simulink model "Upgrade3"  (R2017a)
settings: Solver=FixedStepDiscrete  StartTime=0.0  StopTime=2700000  RelTol=1e-3
model workspace: external: MAT-File upgradeParams.mat (data not in the file)
values from neighbouring files (symbols this model uses):
  ambulance_speed = 60    [upgradeParams.mat]
  delayConstant = 0.25    [upgradeParams.mat]
  hospital_dist = 10    [upgradeParams.mat]
  radius = 15    [upgradeParams.mat]
  transfer_lag = 50    [upgradeParams.mat]
undefined symbols (not defined in the file or in its folder): entity, m, n, readTimer
libraries: sldelib x1
(part 2 of 3)

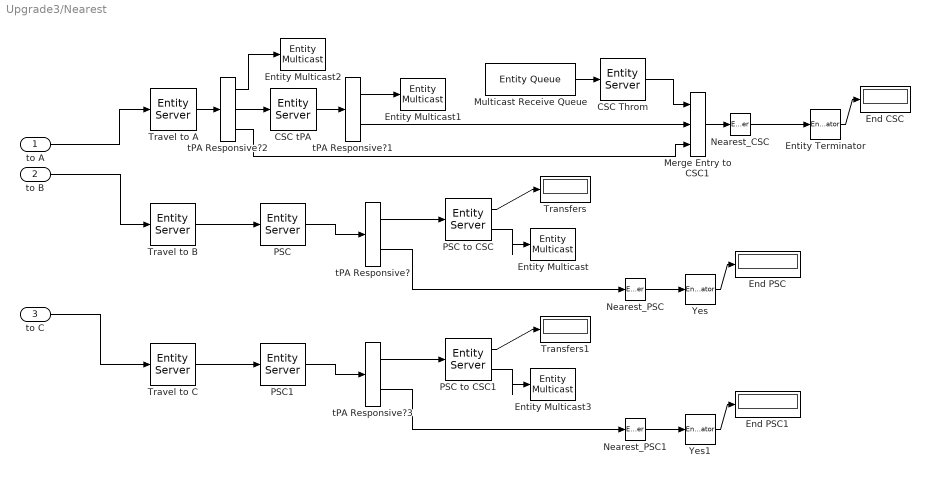
== system Upgrade3/Nearest ==
  to A : Inport
  to B : Inport  Port=2
  to C : Inport  Port=3
  CSC Throm : EntityServer  InputPortMessageModes=m  OutputPortMessageModes=m  Capacity=2  ServiceTimeSource=MATLAB action  ServiceTimeValue=CSC_NTP  ServiceTimeAction=|  ServiceCompleteAction=|
      ServiceTimeAction=|
      | if ~entity.CTA
      |     %did respond to tPA or have hemorrhage
      |     %then only did CTA and discovered no go
      |     if entity.tPA && ((entity.tPAresponse < tPAresp_LVO) | (entity.ICHresp < ICHrate))
      |         dt = CTA_time;
      |     else
      |         dt = CTA_time + CSC_NTP;
      |     end
      | else
      |     dt = CSC_NTP;
      | end
      ServiceCompleteAction=|
      | if ~entity.CTA
      |     entity.CTA=true;
      | end
      | 
      | if entity.throm
      |     %if previously already decided should have thrombectomy
      |     %outcomeType already assigned
      |     entity.thromTime = startTimer() - entity.startTime;
      | elseif ~entity.tPA
      |     %bypassed tPA in CSC
      |     entity.throm = true;
      |     entity.thromTime = startTimer() - entity.startTime;
      |     entity.outcomeType = 3;
      | elseif (entity.tPAresponse >= tPAresp_LVO) && (entity.ICHresp > ICHrate)
      |     %did not respond tPA and did not hemorrhage
      |     entity.throm = true;
      |     entity.thromTime = startTimer() - entity.startTime;
      |     entity.outcomeType = 4;
      | else
      |     %responded to tPA
      |     entity.outcomeType = 2;
      | end
      | 
      | %if had thrombectomy and did not successfully recanalize
      | if entity.throm && entity.thromSuccess > reperf_rate
      |     if entity.outcomeType == 3
      |         entity.outcomeType = 1;
      |     elseif entity.outcomeType == 4
      |         entity.outcomeType = 2;
      |     end
      | end
  CSC tPA : EntityServer  InputPortMessageModes=m  OutputPortMessageModes=m  Capacity=75  ServiceTimeValue=CSC_DTN  ServiceCompleteAction=|
      | entity.tPA = true;
      | entity.tPAtime = startTimer() - entity.startTime;
      | current = entity.tPAtime;
      | 
      | %if has LVO, no throm contraindications, and above min cutoff
      | if entity.LVO && (entity.thromContra > throm_CI) && entity.NIHSS >= throm_min
      |     %don't care if respond to tPA, immediately to thrombectomy
      |     entity.whichPort = 1;
      | else
      |     entity.whichPort = 2;
      |     entity.outcomeType = 2;
      | end
  End CSC : Display
  End PSC : Display
  End PSC1 : Display
  Entity Multicast{,1..3} (4 alike) : EntityMulticast  InputPortMessageModes=m  MulticastTag=Nearest_throm
  Entity Terminator : EntityTerminator  InputPortMessageModes=m  EntryAction=readTimer(entity.totalTime);  NumberEntitiesArrived=on
      settings: OutputPortMap=o0
  Merge Entry to CSC1 : EntityInputSwitch  InputPortMessageModes=m,m,m  OutputPortMessageModes=m  NumberInputPorts=3
      settings: InputPortMap=u1,u2,u3
  Multicast Receive Queue : EntityQueue  OutputPortMessageModes=m  Capacity=100  EntityArrivalSource=Multicast  MulticastTag=Nearest_throm
      settings: OutputPortMap=o5
  Nearest_CSC : EntityServer  InputPortMessageModes=m  OutputPortMessageModes=m  Capacity=inf  ServiceTimeValue=0  EntryAction=|
      | entity.totalTime = startTimer() - entity.startTime;
      | 
      | if entity.LVO
      |     if entity.outcomeType == 1
      |         if entity.totalTime <=360
      |             dist = NT_LVO;
      |         elseif entity.unwitnessed
      |             if entity.totalTime <=960
      |                 dist = MT_DEFUSE3unknown;
      |             else
      |                 dist = MT_DAWNunknown;
      |             end
      |         elseif entity.totalTime <=960
      |             %witnessed and 6-16 hrs
      |             dist = MT_DEFUSE3witnessed;
      |         else
      |             %witnessed and 16-24 hrs
      |             dist = MT_DAWNwitnessed;
      |         end
      |     elseif entity.outcomeType == 2
      |         if entity.tPAtime <=360
      |             dist = tPA_LVO;
      |         else
      |             dist = NT_LVO;
      |         end
      |     elseif entity.outcomeType == 3 | entity.outcomeType ==4
      |         if entity.thromTime <= 180
      |             dist = throm_180;
      |         elseif entity.thromTime <=240
      |             dist = throm_240;
      |         elseif entity.thromTime <=300
      |             dist = throm_300;
      |         elseif entity.thromTime <=360
      |             dist = throm_360;
      |         elseif entity.unwitnessed
      |             if entity.thromTime <=960
      |                 dist = EVT_DEFUSE3unknown;
      |             else
      |                 dist = EVT_DAWNunknown;
      |             end
      |         elseif entity.thromTime <=960
      |             %witnessed and 6-16 hrs
      |             dist = EVT_DEFUSE3witnessed;
      |         else
      |             %witnessed and 16-24 hrs
      |             dist = EVT_DAWNwitnessed;
      |         end
      |     else
      |         dist = [];
      |     end
      | else
      |     if entity.outcomeType==1
      |         if entity.firstArrival <= 90
      |             dist = NT_90;
      |         elseif entity.firstArrival <= 180
      |             dist = NT_180;
      |         elseif entity.firstArrival <= 270
      |             dist = NT_270;
      |         else
      |             dist = NT_360;
      |         end
      |     elseif entity.outcomeType==2
      |         if entity.firstArrival <= 90
      |             dist = tPA_90;
      |         elseif entity.firstArrival <= 180
      |             dist = tPA_180;
      |         elseif entity.firstArrival <= 270
      |             dist = tPA_270;
      |         else
      |             dist = tPA_360;
      |         end
      |     else
      |         dist = [];
      |     end
      | end
      | if isempty(dist)
      |     entity.outcome = 999; %error message basically
      | else
      |     b = find(dist(:)<entity.randOutcome);
      |     if isempty(b)
      |         entity.outcome=0;
      |     else
      |         entity.outcome = b(length(b));
      |     end
      | end
  Nearest_PSC : EntityServer  InputPortMessageModes=m  OutputPortMessageModes=m  Capacity=inf  ServiceTimeValue=0  EntryAction=|
      | entity.totalTime = startTimer() - entity.startTime;
      | 
      | if entity.LVO
      |     if entity.outcomeType == 1
      |         if entity.totalTime <=360
      |             dist = NT_LVO;
      |         elseif entity.unwitnessed
      |             if entity.totalTime <=960
      |                 dist = MT_DEFUSE3unknown;
      |             else
      |                 dist = MT_DAWNunknown;
      |             end
      |         elseif entity.totalTime <=960
      |             %witnessed and 6-16 hrs
      |             dist = MT_DEFUSE3witnessed;
      |         else
      |             %witnessed and 16-24 hrs
      |             dist = MT_DAWNwitnessed;
      |         end
      |     elseif entity.outcomeType == 2
      |         if entity.tPAtime <=360
      |             dist = tPA_LVO;
      |         else
      |             dist = NT_LVO;
      |         end
      |     elseif entity.outcomeType == 3 | entity.outcomeType ==4
      |         if entity.thromTime <= 180
      |             dist = throm_180;
      |         elseif entity.thromTime <=240
      |             dist = throm_240;
      |         elseif entity.thromTime <=300
      |             dist = throm_300;
      |         elseif entity.thromTime <=360
      |             dist = throm_360;
      |         elseif entity.unwitnessed
      |             if entity.thromTime <=960
      |                 dist = EVT_DEFUSE3unknown;
      |             else
      |                 dist = EVT_DAWNunknown;
      |             end
      |         elseif entity.thromTime <=960
      |             %witnessed and 6-16 hrs
      |             dist = EVT_DEFUSE3witnessed;
      |         else
      |             %witnessed and 16-24 hrs
      |             dist = EVT_DAWNwitnessed;
      |         end
      |     else
      |         dist = [];
      |     end
      | else
      |     if entity.outcomeType==1
      |         if entity.firstArrival <= 90
      |             dist = NT_90;
      |         elseif entity.firstArrival <= 180
      |             dist = NT_180;
      |         elseif entity.firstArrival <= 270
      |             dist = NT_270;
      |         else
      |             dist = NT_360;
      |         end
      |     elseif entity.outcomeType==2
      |         if entity.firstArrival <= 90
      |             dist = tPA_90;
      |         elseif entity.firstArrival <= 180
      |             dist = tPA_180;
      |         elseif entity.firstArrival <= 270
      |             dist = tPA_270;
      |         else
      |             dist = tPA_360;
      |         end
      |     else
      |         dist = [];
      |     end
      | end
      | if isempty(dist)
      |     entity.outcome = 999; %error message basically
      | else
      |     b = find(dist(:)<entity.randOutcome);
      |     if isempty(b)
      |         entity.outcome=0;
      |     else
      |         entity.outcome = b(length(b));
      |     end
      | end
  Nearest_PSC1 : EntityServer  InputPortMessageModes=m  OutputPortMessageModes=m  Capacity=inf  ServiceTimeValue=0  EntryAction=|
      | entity.totalTime = startTimer() - entity.startTime;
      | 
      | if entity.LVO
      |     if entity.outcomeType == 1
      |         if entity.totalTime <=360
      |             dist = NT_LVO;
      |         elseif entity.unwitnessed
      |             if entity.totalTime <=960
      |                 dist = MT_DEFUSE3unknown;
      |             else
      |                 dist = MT_DAWNunknown;
      |             end
      |         elseif entity.totalTime <=960
      |             %witnessed and 6-16 hrs
      |             dist = MT_DEFUSE3witnessed;
      |         else
      |             %witnessed and 16-24 hrs
      |             dist = MT_DAWNwitnessed;
      |         end
      |     elseif entity.outcomeType == 2
      |         if entity.tPAtime <=360
      |             dist = tPA_LVO;
      |         else
      |             dist = NT_LVO;
      |         end
      |     elseif entity.outcomeType == 3 | entity.outcomeType ==4
      |         if entity.thromTime <= 180
      |             dist = throm_180;
      |         elseif entity.thromTime <=240
      |             dist = throm_240;
      |         elseif entity.thromTime <=300
      |             dist = throm_300;
      |         elseif entity.thromTime <=360
      |             dist = throm_360;
      |         elseif entity.unwitnessed
      |             if entity.thromTime <=960
      |                 dist = EVT_DEFUSE3unknown;
      |             else
      |                 dist = EVT_DAWNunknown;
      |             end
      |         elseif entity.thromTime <=960
      |             %witnessed and 6-16 hrs
      |             dist = EVT_DEFUSE3witnessed;
      |         else
      |             %witnessed and 16-24 hrs
      |             dist = EVT_DAWNwitnessed;
      |         end
      |     else
      |         dist = [];
      |     end
      | else
      |     if entity.outcomeType==1
      |         if entity.firstArrival <= 90
      |             dist = NT_90;
      |         elseif entity.firstArrival <= 180
      |             dist = NT_180;
      |         elseif entity.firstArrival <= 270
      |             dist = NT_270;
      |         else
      |             dist = NT_360;
      |         end
      |     elseif entity.outcomeType==2
      |         if entity.firstArrival <= 90
      |             dist = tPA_90;
      |         elseif entity.firstArrival <= 180
      |             dist = tPA_180;
      |         elseif entity.firstArrival <= 270
      |             dist = tPA_270;
      |         else
      |             dist = tPA_360;
      |         end
      |     else
      |         dist = [];
      |     end
      | end
      | if isempty(dist)
      |     entity.outcome = 999; %error message basically
      | else
      |     b = find(dist(:)<entity.randOutcome);
      |     if isempty(b)
      |         entity.outcome=0;
      |     else
      |         entity.outcome = b(length(b));
      |     end
      | end
  PSC : EntityServer  InputPortMessageModes=m  OutputPortMessageModes=m  Capacity=50  ServiceTimeSource=MATLAB action  ServiceTimeValue=PSC_DTN  ServiceTimeAction=|  ServiceCompleteAction=|
      ServiceTimeAction=|
      | %no contraindications for tPA
      | if entity.tPAcontra > tPA_CI && (entity.firstArrival <= tPA_cutoff)
      |     if entity.LVO && PSC_CTA && (entity.tPAresponse > tPAresp_LVO) && (entity.ICHresp > ICHrate)
      |         dt = PSC_DTN + CTA_time;
      |     else
      |         dt = PSC_DTN;
      |     end
      | else
      |     if entity.LVO && PSC_CTA
      |         dt = CTA_time;
      |     else
      |         dt = 0;
      |     end
      | end
      ServiceCompleteAction=|
      | current = startTimer() - entity.startTime;
      | 
      | %get tPA if no contraindications and less than 4.5 hours
      | if (entity.tPAcontra > tPA_CI) && (entity.firstArrival <= tPA_cutoff)
      |     entity.tPA = true;
      |     entity.tPAtime = startTimer() - entity.startTime;
      |     if entity.LVO && (entity.thromContra > throm_CI) && (entity.tPAresponse > tPAresp_LVO) && (entity.ICHresp > ICHrate) && entity.NIHSS >= throm_min
      |         %has LVO, didn't respond to tPA, no contraindications, no hemorrhage, above min NIHSS
      |         entity.whichPort = 1;
      |         entity.outcomeType = 4;
      |         entity.throm = true;
      |     else
      |         %no LVO, responded to tPA, hemorrhaged or has throm contraindications
      |         entity.whichPort = 2;
      |         entity.outcomeType = 2;
      |     end
      | else    
      | %no tPA
      |     if entity.LVO && (entity.NIHSS >= throm_min) && (((current + hospital_dist <= HERMES_cutoff) && (entity.thromContra > throm_CI)) | ((current + hospital_dist <= DEFUSE_cutoff) && (entity.DAWN <= DEFUSEe)) | ((current + hospital_dist <= DAWN_cutoff) && (entity.DAWN <= DAWNe) && (entity.NIHSS >= DAWN_NIHSS_min)))
      |         %ineligible for tPA but still eligible for thrombectomy
      |         entity.whichPort = 1;
      |         entity.outcomeType = 3;
      |         entity.throm = true;    
      |     else
      |     %no treatment
      |         entity.whichPort = 2;
      |         entity.outcomeType = 1;
      |     end
      | end
      | 
      | if PSC_CTA
      |     entity.CTA=true;
      | end
  PSC to CSC : EntityServer  InputPortMessageModes=m  OutputPortMessageModes=n,m  Capacity=75  ServiceTimeValue=((hospital_dist/ambulance_speed)*60)+transfer_lag  ServiceCompleteAction=|  NumberEntitiesDeparted=on
      | entity.throm = true;
      | entity.transfer = true;
      settings: OutputPortMap=o0,o9
  PSC to CSC1 : EntityServer  InputPortMessageModes=m  OutputPortMessageModes=n,m  Capacity=75  ServiceTimeValue=((hospital_dist/ambulance_speed)*60)+transfer_lag  ServiceCompleteAction=|  NumberEntitiesDeparted=on
      | entity.throm = true;
      | entity.transfer = true;
      settings: OutputPortMap=o0,o9
  PSC1 : EntityServer  InputPortMessageModes=m  OutputPortMessageModes=m  Capacity=50  ServiceTimeSource=MATLAB action  ServiceTimeValue=PSC_DTN  ServiceTimeAction=|  ServiceCompleteAction=|
      ServiceTimeAction=|
      | %no contraindications for tPA
      | if entity.tPAcontra > tPA_CI && (entity.firstArrival <= tPA_cutoff)
      |     if entity.LVO && PSC_CTA && (entity.tPAresponse > tPAresp_LVO) && (entity.ICHresp > ICHrate)
      |         dt = PSC_DTN + CTA_time;
      |     else
      |         dt = PSC_DTN;
      |     end
      | else
      |     if entity.LVO && PSC_CTA
      |         dt = CTA_time;
      |     else
      |         dt = 0;
      |     end
      | end
      ServiceCompleteAction=|
      | current = startTimer() - entity.startTime;
      | 
      | %get tPA if no contraindications and less than 4.5 hours
      | if (entity.tPAcontra > tPA_CI) && (entity.firstArrival <= tPA_cutoff)
      |     entity.tPA = true;
      |     entity.tPAtime = startTimer() - entity.startTime;
      |     if entity.LVO && (entity.thromContra > throm_CI) && (entity.tPAresponse > tPAresp_LVO) && (entity.ICHresp > ICHrate) && entity.NIHSS >= throm_min
      |         %has LVO, didn't respond to tPA, no contraindications, no hemorrhage, above min NIHSS
      |         entity.whichPort = 1;
      |         entity.outcomeType = 4;
      |         entity.throm = true;
      |     else
      |         %no LVO, responded to tPA, hemorrhaged or has throm contraindications
      |         entity.whichPort = 2;
      |         entity.outcomeType = 2;
      |     end
      | else    
      | %no tPA
      |     if entity.LVO && (entity.NIHSS >= throm_min) && (((current + hospital_dist <= HERMES_cutoff) && (entity.thromContra > throm_CI)) | ((current + hospital_dist <= DEFUSE_cutoff) && (entity.DAWN <= DEFUSEe)) | ((current + hospital_dist <= DAWN_cutoff) && (entity.DAWN <= DAWNe) && (entity.NIHSS >= DAWN_NIHSS_min)))
      |         %ineligible for tPA but still eligible for thrombectomy
      |         entity.whichPort = 1;
      |         entity.outcomeType = 3;
      |         entity.throm = true;    
      |     else
      |     %no treatment
      |         entity.whichPort = 2;
      |         entity.outcomeType = 1;
      |     end
      | end
      | 
      | if PSC_CTA
      |     entity.CTA=true;
      | end
  Transfers : Display
  Transfers1 : Display
  Travel to A : EntityServer  InputPortMessageModes=m  OutputPortMessageModes=m  Capacity=75  ServiceTimeSource=Attribute  ServiceTimeValue=cscDis  ServiceTimeAttributeName=aDistance  EntryAction=entity.firstHosp = 1;  ServiceCompleteAction=|
      | %time exceeds 4.5 hours then bypass tPA
      | %exceeds 24 hours then no thrombectomy
      | current = startTimer()-entity.startTime;
      | 
      | %past 24 hours
      | if current >= DAWN_cutoff
      |     entity.whichPort = 3;
      |     entity.outcomeType = 1;
      | %past 4.5 hrs or have contraindications, no tPA
      | elseif (current >= tPA_cutoff) | (entity.tPAcontra < tPA_CI)
      |     if entity.LVO && entity.NIHSS >= throm_min && (((current <= HERMES_cutoff) && (entity.thromContra > throm_CI)) | ((current <= DEFUSE_cutoff) && (entity.DAWN <= DEFUSEe)) | ((current <= DAWN_cutoff) && (entity.DAWN <= DAWNe) && (entity.NIHSS >= DAWN_NIHSS_min)))
      |         %with LVO, no CI for thrombectomy, above min NIHSS cutoff
      |         entity.whichPort = 1;
      |         entity.throm = true;
      |         entity.outcomeType = 3;
      |     else
      |         %not eligible for tPA or thrombectomy
      |         entity.whichPort = 3;
      |         entity.outcomeType = 1;
      |     end
      | else
      |     entity.whichPort = 2;
      | end
      | 
      | entity.firstArrival = startTimer() - entity.startTime;
  Travel to B : EntityServer  InputPortMessageModes=m  OutputPortMessageModes=m  Capacity=75  ServiceTimeSource=Attribute  ServiceTimeValue=9  ServiceTimeAttributeName=bDistance  EntryAction=entity.firstHosp = 2;  ServiceCompleteAction=entity.firstArrival = startTimer() - entity.startTime;
  Travel to C : EntityServer  InputPortMessageModes=m  OutputPortMessageModes=m  Capacity=75  ServiceTimeSource=Attribute  ServiceTimeValue=9  ServiceTimeAttributeName=cDistance  EntryAction=entity.firstHosp = 3;  ServiceCompleteAction=entity.firstArrival = startTimer() - entity.startTime;
  Yes : EntityTerminator  InputPortMessageModes=m  EntryAction=readTimer(entity.totalTime);  NumberEntitiesArrived=on
      settings: OutputPortMap=o0
  Yes1 : EntityTerminator  InputPortMessageModes=m  EntryAction=readTimer(entity.totalTime);  NumberEntitiesArrived=on
      settings: OutputPortMap=o0
  tPA Responsive? : EntityOutputSwitch  InputPortMessageModes=m  OutputPortMessageModes=m,m  SwitchingCriterion=From attribute  SwitchAttributeName=whichPort
  tPA Responsive?1 : EntityOutputSwitch  InputPortMessageModes=m  OutputPortMessageModes=m,m  SwitchingCriterion=From attribute  SwitchAttributeName=whichPort
  tPA Responsive?2 : EntityOutputSwitch  InputPortMessageModes=m  OutputPortMessageModes=m,m,m  NumberOutputPorts=3  SwitchingCriterion=From attribute  SwitchAttributeName=whichPort
      settings: OutputPortMap=o0,o1,o2
  tPA Responsive?3 : EntityOutputSwitch  InputPortMessageModes=m  OutputPortMessageModes=m,m  SwitchingCriterion=From attribute  SwitchAttributeName=whichPort
  wires:
  to B/1 -> Travel to B/1
  to A/1 -> Travel to A/1
  tPA Responsive?/1 -> PSC to CSC/1
  PSC/1 -> tPA Responsive?/1
  PSC to CSC/1 -> Transfers/1
  Yes/1 -> End PSC/1
  Entity Terminator/1 -> End CSC/1
  CSC tPA/1 -> tPA Responsive?1/1
  CSC Throm/1 -> Merge Entry to CSC1/1
  PSC to CSC/2 -> Entity Multicast/1
  tPA Responsive?1/1 -> Entity Multicast1/1
  Multicast Receive Queue/1 -> CSC Throm/1
  tPA Responsive?1/2 -> Merge Entry to CSC1/2
  Travel to A/1 -> tPA Responsive?2/1
  tPA Responsive?2/1 -> Entity Multicast2/1
  tPA Responsive?2/2 -> CSC tPA/1
  tPA Responsive?2/3 -> Merge Entry to CSC1/3
  Merge Entry to CSC1/1 -> Nearest_CSC/1
  Nearest_CSC/1 -> Entity Terminator/1
  Travel to B/1 -> PSC/1
  Nearest_PSC/1 -> Yes/1
  tPA Responsive?/2 -> Nearest_PSC/1
  Travel to C/1 -> PSC1/1
  PSC to CSC1/2 -> Entity Multicast3/1
  tPA Responsive?3/2 -> Nearest_PSC1/1
  Yes1/1 -> End PSC1/1
  tPA Responsive?3/1 -> PSC to CSC1/1
  Nearest_PSC1/1 -> Yes1/1
  PSC to CSC1/1 -> Transfers1/1
  PSC1/1 -> tPA Responsive?3/1
  to C/1 -> Travel to C/1

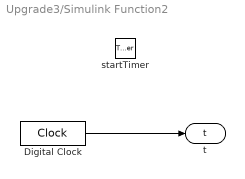
== system Upgrade3/Simulink Function2 ==
  startTimer : TriggerPort  TriggerType=function-call  IsSimulinkFunction=on  FunctionName=startTimer  VariantControl=Variant
  Digital Clock : DigitalClock  SampleTime=-1
  t : ArgOut  DisableCoverage=on  ArgumentName=t
  wires:
  Digital Clock/1 -> t/1

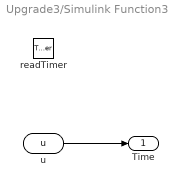
== system Upgrade3/Simulink Function3 ==
  readTimer : TriggerPort  TriggerType=function-call  IsSimulinkFunction=on  FunctionName=readTimer  VariantControl=Variant
  u : ArgIn  DisableCoverage=on  ArgumentName=u
  Time : Outport
  wires:
  u/1 -> Time/1

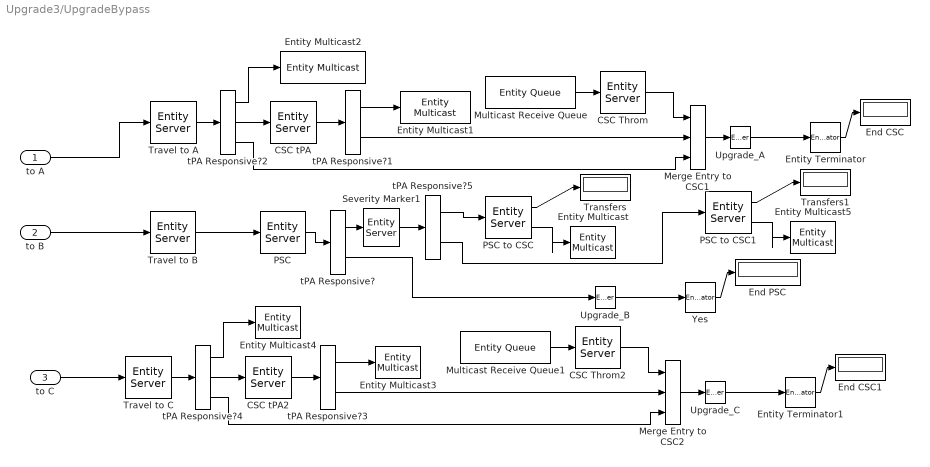
== system Upgrade3/UpgradeBypass ==
  to A : Inport
  to B : Inport  Port=2
  to C : Inport  Port=3
  CSC Throm : EntityServer  InputPortMessageModes=m  OutputPortMessageModes=m  Capacity=2  ServiceTimeSource=MATLAB action  ServiceTimeValue=CSC_NTP  ServiceTimeAction=|  ServiceCompleteAction=|
      ServiceTimeAction=|
      | if ~entity.CTA
      |     %did respond to tPA or have hemorrhage
      |     %then only did CTA and discovered no go
      |     if entity.tPA && ((entity.tPAresponse < tPAresp_LVO) | (entity.ICHresp < ICHrate))
      |         dt = CTA_time;
      |     else
      |         dt = CTA_time + CSC_NTP;
      |     end
      | else
      |     dt = CSC_NTP;
      | end
      ServiceCompleteAction=|
      | if ~entity.CTA
      |     entity.CTA=true;
      | end
      | 
      | if entity.throm
      |     %if previously already decided should have thrombectomy
      |     %outcomeType already assigned
      |     entity.thromTime = startTimer() - entity.startTime;
      | elseif ~entity.tPA
      |     %bypassed tPA in CSC
      |     entity.throm = true;
      |     entity.thromTime = startTimer() - entity.startTime;
      |     entity.outcomeType = 3;
      | elseif (entity.tPAresponse >= tPAresp_LVO) && (entity.ICHresp > ICHrate)
      |     %did not respond tPA and did not hemorrhage
      |     entity.throm = true;
      |     entity.thromTime = startTimer() - entity.startTime;
      |     entity.outcomeType = 4;
      | else
      |     %responded to tPA
      |     entity.outcomeType = 2;
      | end
      | 
      | %if had thrombectomy and did not successfully recanalize
      | if entity.throm && entity.thromSuccess > reperf_rate
      |     if entity.outcomeType == 3
      |         entity.outcomeType = 1;
      |     elseif entity.outcomeType == 4
      |         entity.outcomeType = 2;
      |     end
      | end
  CSC Throm2 : EntityServer  InputPortMessageModes=m  OutputPortMessageModes=m  Capacity=2  ServiceTimeSource=MATLAB action  ServiceTimeValue=CSC_NTP  ServiceTimeAction=|  ServiceCompleteAction=|
      ServiceTimeAction=|
      | if ~entity.CTA
      |     %did respond to tPA or have hemorrhage
      |     %then only did CTA and discovered no go
      |     if entity.tPA && ((entity.tPAresponse < tPAresp_LVO) | (entity.ICHresp < ICHrate))
      |         dt = CTA_time;
      |     else
      |         dt = CTA_time + CSC_NTP;
      |     end
      | else
      |     dt = CSC_NTP;
      | end
      ServiceCompleteAction=|
      | if ~entity.CTA
      |     entity.CTA=true;
      | end
      | 
      | if entity.throm
      |     %if previously already decided should have thrombectomy
      |     %outcomeType already assigned
      |     entity.thromTime = startTimer() - entity.startTime;
      | elseif ~entity.tPA
      |     %bypassed tPA in CSC
      |     entity.throm = true;
      |     entity.thromTime = startTimer() - entity.startTime;
      |     entity.outcomeType = 3;
      | elseif (entity.tPAresponse >= tPAresp_LVO) && (entity.ICHresp > ICHrate)
      |     %did not respond tPA and did not hemorrhage
      |     entity.throm = true;
      |     entity.thromTime = startTimer() - entity.startTime;
      |     entity.outcomeType = 4;
      | else
      |     %responded to tPA
      |     entity.outcomeType = 2;
      | end
      | 
      | %if had thrombectomy and did not successfully recanalize
      | if entity.throm && entity.thromSuccess > reperf_rate
      |     if entity.outcomeType == 3
      |         entity.outcomeType = 1;
      |     elseif entity.outcomeType == 4
      |         entity.outcomeType = 2;
      |     end
      | end
  CSC tPA : EntityServer  InputPortMessageModes=m  OutputPortMessageModes=m  Capacity=75  ServiceTimeValue=CSC_DTN  ServiceCompleteAction=|
      | entity.tPA = true;
      | entity.tPAtime = startTimer() - entity.startTime;
      | current = entity.tPAtime;
      | 
      | %if has LVO, no throm contraindications, and above min cutoff
      | if entity.LVO && (entity.thromContra > throm_CI) && entity.NIHSS >= throm_min
      |     %don't care if respond to tPA, immediately to thrombectomy
      |     entity.whichPort = 1;
      | else
      |     entity.whichPort = 2;
      |     entity.outcomeType = 2;
      | end
  CSC tPA2 : EntityServer  InputPortMessageModes=m  OutputPortMessageModes=m  Capacity=75  ServiceTimeValue=CSC_DTN  ServiceCompleteAction=|
      | entity.tPA = true;
      | entity.tPAtime = startTimer() - entity.startTime;
      | current = entity.tPAtime;
      | 
      | %if has LVO, no throm contraindications, and above min cutoff
      | if entity.LVO && (entity.thromContra > throm_CI) && entity.NIHSS >= throm_min
      |     %don't care if respond to tPA, immediately to thrombectomy
      |     entity.whichPort = 1;
      | else
      |     entity.whichPort = 2;
      |     entity.outcomeType = 2;
      | end
  End CSC : Display
  End CSC1 : Display
  End PSC : Display
  Entity Multicast : EntityMulticast  InputPortMessageModes=m  MulticastTag=UpgradeRI_throm1
  Entity Multicast1 : EntityMulticast  InputPortMessageModes=m  MulticastTag=UpgradeRI_throm1
  Entity Multicast2 : EntityMulticast  InputPortMessageModes=m  MulticastTag=UpgradeRI_throm1
  Entity Multicast3 : EntityMulticast  InputPortMessageModes=m  MulticastTag=UpgradeRI_throm2
  Entity Multicast4 : EntityMulticast  InputPortMessageModes=m  MulticastTag=UpgradeRI_throm2
  Entity Multicast5 : EntityMulticast  InputPortMessageModes=m  MulticastTag=UpgradeRI_throm2
  Entity Terminator : EntityTerminator  InputPortMessageModes=m  EntryAction=readTimer(entity.totalTime);  NumberEntitiesArrived=on
      settings: OutputPortMap=o0
  Entity Terminator1 : EntityTerminator  InputPortMessageModes=m  EntryAction=readTimer(entity.totalTime);  NumberEntitiesArrived=on
      settings: OutputPortMap=o0
  Merge Entry to CSC1 : EntityInputSwitch  InputPortMessageModes=m,m,m  OutputPortMessageModes=m  NumberInputPorts=3
      settings: InputPortMap=u1,u2,u3
  Merge Entry to CSC2 : EntityInputSwitch  InputPortMessageModes=m,m,m  OutputPortMessageModes=m  NumberInputPorts=3
      settings: InputPortMap=u1,u2,u3
  Multicast Receive Queue : EntityQueue  OutputPortMessageModes=m  Capacity=100  EntityArrivalSource=Multicast  MulticastTag=UpgradeRI_throm1
      settings: OutputPortMap=o5
  Multicast Receive Queue1 : EntityQueue  OutputPortMessageModes=m  Capacity=100  EntityArrivalSource=Multicast  MulticastTag=UpgradeRI_throm2
      settings: OutputPortMap=o5
  PSC : EntityServer  InputPortMessageModes=m  OutputPortMessageModes=m  Capacity=50  ServiceTimeSource=MATLAB action  ServiceTimeValue=PSC_DTN  ServiceTimeAction=|  ServiceCompleteAction=|
      ServiceTimeAction=|
      | %no contraindications for tPA
      | if entity.tPAcontra > tPA_CI && (entity.firstArrival <= tPA_cutoff)
      |     if entity.LVO && PSC_CTA && (entity.tPAresponse > tPAresp_LVO) && (entity.ICHresp > ICHrate)
      |         dt = PSC_DTN + CTA_time;
      |     else
      |         dt = PSC_DTN;
      |     end
      | else
      |     if entity.LVO && PSC_CTA
      |         dt = CTA_time;
      |     else
      |         dt = 0;
      |     end
      | end
      ServiceCompleteAction=|
      | current = startTimer() - entity.startTime;
      | 
      | %get tPA if no contraindications and less than 4.5 hours
      | if (entity.tPAcontra > tPA_CI) && (entity.firstArrival <= tPA_cutoff)
      |     entity.tPA = true;
      |     entity.tPAtime = startTimer() - entity.startTime;
      |     if entity.LVO && (entity.thromContra > throm_CI) && (entity.tPAresponse > tPAresp_LVO) && (entity.ICHresp > ICHrate) && entity.NIHSS >= throm_min
      |         %has LVO, didn't respond to tPA, no contraindications, no hemorrhage, above min NIHSS
      |         entity.whichPort = 1;
      |         entity.outcomeType = 4;
      |         entity.throm = true;
      |     else
      |         %no LVO, responded to tPA, hemorrhaged or has throm contraindications
      |         entity.whichPort = 2;
      |         entity.outcomeType = 2;
      |     end
      | else    
      | %no tPA
      |     if entity.LVO && (entity.NIHSS >= throm_min) && (((current + hospital_dist <= HERMES_cutoff) && (entity.thromContra > throm_CI)) | ((current + hospital_dist <= DEFUSE_cutoff) && (entity.DAWN <= DEFUSEe)) | ((current + hospital_dist <= DAWN_cutoff) && (entity.DAWN <= DAWNe) && (entity.NIHSS >= DAWN_NIHSS_min)))
      |         %ineligible for tPA but still eligible for thrombectomy
      |         entity.whichPort = 1;
      |         entity.outcomeType = 3;
      |         entity.throm = true;    
      |     else
      |     %no treatment
      |         entity.whichPort = 2;
      |         entity.outcomeType = 1;
      |     end
      | end
      | 
      | if PSC_CTA
      |     entity.CTA=true;
      | end
  PSC to CSC : EntityServer  InputPortMessageModes=m  OutputPortMessageModes=n,m  Capacity=75  ServiceTimeValue=((hospital_dist/ambulance_speed)*60)+transfer_lag  ServiceCompleteAction=|  NumberEntitiesDeparted=on
      | entity.throm = true;
      | entity.transfer = true;
      settings: OutputPortMap=o0,o9
  PSC to CSC1 : EntityServer  InputPortMessageModes=m  OutputPortMessageModes=n,m  Capacity=75  ServiceTimeValue=((hospital_dist/ambulance_speed)*60)+transfer_lag  ServiceCompleteAction=|  NumberEntitiesDeparted=on
      | entity.throm = true;
      | entity.transfer = true;
      settings: OutputPortMap=o0,o9
  Severity Marker1 : EntityServer  InputPortMessageModes=m  OutputPortMessageModes=m  Capacity=50  ServiceTimeValue=0  ServiceTimeAttributeName=onset  EntryAction=entity.whichPort = randi(2);
  Transfers : Display
  Transfers1 : Display
  Travel to A : EntityServer  InputPortMessageModes=m  OutputPortMessageModes=m  Capacity=75  ServiceTimeSource=Attribute  ServiceTimeValue=cscDis  ServiceTimeAttributeName=aDistance  EntryAction=entity.firstHosp = 1;  ServiceCompleteAction=|
      | %time exceeds 4.5 hours then bypass tPA
      | %exceeds 24 hours then no thrombectomy
      | current = startTimer()-entity.startTime;
      | 
      | %past 24 hours
      | if current >= DAWN_cutoff
      |     entity.whichPort = 3;
      |     entity.outcomeType = 1;
      | %past 4.5 hrs or have contraindications, no tPA
      | elseif (current >= tPA_cutoff) | (entity.tPAcontra < tPA_CI)
      |     if entity.LVO && entity.NIHSS >= throm_min && (((current <= HERMES_cutoff) && (entity.thromContra > throm_CI)) | ((current <= DEFUSE_cutoff) && (entity.DAWN <= DEFUSEe)) | ((current <= DAWN_cutoff) && (entity.DAWN <= DAWNe) && (entity.NIHSS >= DAWN_NIHSS_min)))
      |         %with LVO, no CI for thrombectomy, above min NIHSS cutoff
      |         entity.whichPort = 1;
      |         entity.throm = true;
      |         entity.outcomeType = 3;
      |     else
      |         %not eligible for tPA or thrombectomy
      |         entity.whichPort = 3;
      |         entity.outcomeType = 1;
      |     end
      | else
      |     entity.whichPort = 2;
      | end
      | 
      | entity.firstArrival = startTimer() - entity.startTime;
  Travel to B : EntityServer  InputPortMessageModes=m  OutputPortMessageModes=m  Capacity=75  ServiceTimeSource=Attribute  ServiceTimeValue=9  ServiceTimeAttributeName=bDistance  EntryAction=entity.firstHosp = 2;  ServiceCompleteAction=entity.firstArrival = startTimer() - entity.startTime;
  Travel to C : EntityServer  InputPortMessageModes=m  OutputPortMessageModes=m  Capacity=75  ServiceTimeSource=Attribute  ServiceTimeValue=cscDis  ServiceTimeAttributeName=cDistance  EntryAction=entity.firstHosp = 3;  ServiceCompleteAction=|
      | %time exceeds 4.5 hours then bypass tPA
      | %exceeds 24 hours then no thrombectomy
      | current = startTimer()-entity.startTime;
      | 
      | %past 24 hours
      | if current >= DAWN_cutoff
      |     entity.whichPort = 3;
      |     entity.outcomeType = 1;
      | %past 4.5 hrs or have contraindications, no tPA
      | elseif (current >= tPA_cutoff) | (entity.tPAcontra < tPA_CI)
      |     if entity.LVO && entity.NIHSS >= throm_min && (((current <= HERMES_cutoff) && (entity.thromContra > throm_CI)) | ((current <= DEFUSE_cutoff) && (entity.DAWN <= DEFUSEe)) | ((current <= DAWN_cutoff) && (entity.DAWN <= DAWNe) && (entity.NIHSS >= DAWN_NIHSS_min)))
      |         %with LVO, no CI for thrombectomy, above min NIHSS cutoff
      |         entity.whichPort = 1;
      |         entity.throm = true;
      |         entity.outcomeType = 3;
      |     else
      |         %not eligible for tPA or thrombectomy
      |         entity.whichPort = 3;
      |         entity.outcomeType = 1;
      |     end
      | else
      |     entity.whichPort = 2;
      | end
      | 
      | entity.firstArrival = startTimer() - entity.startTime;
  Upgrade_A : EntityServer  InputPortMessageModes=m  OutputPortMessageModes=m  Capacity=inf  ServiceTimeValue=0  EntryAction=|
      | entity.totalTime = startTimer() - entity.startTime;
      | 
      | if entity.LVO
      |     if entity.outcomeType == 1
      |         if entity.totalTime <=360
      |             dist = NT_LVO;
      |         elseif entity.unwitnessed
      |             if entity.totalTime <=960
      |                 dist = MT_DEFUSE3unknown;
      |             else
      |                 dist = MT_DAWNunknown;
      |             end
      |         elseif entity.totalTime <=960
      |             %witnessed and 6-16 hrs
      |             dist = MT_DEFUSE3witnessed;
      |         else
      |             %witnessed and 16-24 hrs
      |             dist = MT_DAWNwitnessed;
      |         end
      |     elseif entity.outcomeType == 2
      |         if entity.tPAtime <=360
      |             dist = tPA_LVO;
      |         else
      |             dist = NT_LVO;
      |         end
      |     elseif entity.outcomeType == 3 | entity.outcomeType ==4
      |         if entity.thromTime <= 180
      |             dist = throm_180;
      |         elseif entity.thromTime <=240
      |             dist = throm_240;
      |         elseif entity.thromTime <=300
      |             dist = throm_300;
      |         elseif entity.thromTime <=360
      |             dist = throm_360;
      |         elseif entity.unwitnessed
      |             if entity.thromTime <=960
      |                 dist = EVT_DEFUSE3unknown;
      |             else
      |                 dist = EVT_DAWNunknown;
      |             end
      |         elseif entity.thromTime <=960
      |             %witnessed and 6-16 hrs
      |             dist = EVT_DEFUSE3witnessed;
      |         else
      |             %witnessed and 16-24 hrs
      |             dist = EVT_DAWNwitnessed;
      |         end
      |     else
      |         dist = [];
      |     end
      | else
      |     if entity.outcomeType==1
      |         if entity.firstArrival <= 90
      |             dist = NT_90;
      |         elseif entity.firstArrival <= 180
      |             dist = NT_180;
      |         elseif entity.firstArrival <= 270
      |             dist = NT_270;
      |         else
      |             dist = NT_360;
      |         end
      |     elseif entity.outcomeType==2
      |         if entity.firstArrival <= 90
      |             dist = tPA_90;
      |         elseif entity.firstArrival <= 180
      |             dist = tPA_180;
      |         elseif entity.firstArrival <= 270
      |             dist = tPA_270;
      |         else
      |             dist = tPA_360;
      |         end
      |     else
      |         dist = [];
      |     end
      | end
      | if isempty(dist)
      |     entity.outcome = 999; %error message basically
      | else
      |     b = find(dist(:)<entity.randOutcome);
      |     if isempty(b)
      |         entity.outcome=0;
      |     else
      |         entity.outcome = b(length(b));
      |     end
      | end
  Upgrade_B : EntityServer  InputPortMessageModes=m  OutputPortMessageModes=m  Capacity=inf  ServiceTimeValue=0  EntryAction=|
      | entity.totalTime = startTimer() - entity.startTime;
      | 
      | if entity.LVO
      |     if entity.outcomeType == 1
      |         if entity.totalTime <=360
      |             dist = NT_LVO;
      |         elseif entity.unwitnessed
      |             if entity.totalTime <=960
      |                 dist = MT_DEFUSE3unknown;
      |             else
      |                 dist = MT_DAWNunknown;
      |             end
      |         elseif entity.totalTime <=960
      |             %witnessed and 6-16 hrs
      |             dist = MT_DEFUSE3witnessed;
      |         else
      |             %witnessed and 16-24 hrs
      |             dist = MT_DAWNwitnessed;
      |         end
      |     elseif entity.outcomeType == 2
      |         if entity.tPAtime <=360
      |             dist = tPA_LVO;
      |         else
      |             dist = NT_LVO;
      |         end
      |     elseif entity.outcomeType == 3 | entity.outcomeType ==4
      |         if entity.thromTime <= 180
      |             dist = throm_180;
      |         elseif entity.thromTime <=240
      |             dist = throm_240;
      |         elseif entity.thromTime <=300
      |             dist = throm_300;
      |         elseif entity.thromTime <=360
      |             dist = throm_360;
      |         elseif entity.unwitnessed
      |             if entity.thromTime <=960
      |                 dist = EVT_DEFUSE3unknown;
      |             else
      |                 dist = EVT_DAWNunknown;
      |             end
      |         elseif entity.thromTime <=960
      |             %witnessed and 6-16 hrs
      |             dist = EVT_DEFUSE3witnessed;
      |         else
      |             %witnessed and 16-24 hrs
      |             dist = EVT_DAWNwitnessed;
      |         end
      |     else
      |         dist = [];
      |     end
      | else
      |     if entity.outcomeType==1
      |         if entity.firstArrival <= 90
      |             dist = NT_90;
      |         elseif entity.firstArrival <= 180
      |             dist = NT_180;
      |         elseif entity.firstArrival <= 270
      |             dist = NT_270;
      |         else
      |             dist = NT_360;
      |         end
      |     elseif entity.outcomeType==2
      |         if entity.firstArrival <= 90
      |             dist = tPA_90;
      |         elseif entity.firstArrival <= 180
      |             dist = tPA_180;
      |         elseif entity.firstArrival <= 270
      |             dist = tPA_270;
      |         else
      |             dist = tPA_360;
      |         end
      |     else
      |         dist = [];
      |     end
      | end
      | if isempty(dist)
      |     entity.outcome = 999; %error message basically
      | else
      |     b = find(dist(:)<entity.randOutcome);
      |     if isempty(b)
      |         entity.outcome=0;
      |     else
      |         entity.outcome = b(length(b));
      |     end
      | end
  Upgrade_C : EntityServer  InputPortMessageModes=m  OutputPortMessageModes=m  Capacity=inf  ServiceTimeValue=0  EntryAction=|
      | entity.totalTime = startTimer() - entity.startTime;
      | 
      | if entity.LVO
      |     if entity.outcomeType == 1
      |         if entity.totalTime <=360
      |             dist = NT_LVO;
      |         elseif entity.unwitnessed
      |             if entity.totalTime <=960
      |                 dist = MT_DEFUSE3unknown;
      |             else
      |                 dist = MT_DAWNunknown;
      |             end
      |         elseif entity.totalTime <=960
      |             %witnessed and 6-16 hrs
      |             dist = MT_DEFUSE3witnessed;
      |         else
      |             %witnessed and 16-24 hrs
      |             dist = MT_DAWNwitnessed;
      |         end
      |     elseif entity.outcomeType == 2
      |         if entity.tPAtime <=360
      |             dist = tPA_LVO;
      |         else
      |             dist = NT_LVO;
      |         end
      |     elseif entity.outcomeType == 3 | entity.outcomeType ==4
      |         if entity.thromTime <= 180
      |             dist = throm_180;
      |         elseif entity.thromTime <=240
      |             dist = throm_240;
      |         elseif entity.thromTime <=300
      |             dist = throm_300;
      |         elseif entity.thromTime <=360
      |             dist = throm_360;
      |         elseif entity.unwitnessed
      |             if entity.thromTime <=960
      |                 dist = EVT_DEFUSE3unknown;
      |             else
      |                 dist = EVT_DAWNunknown;
      |             end
      |         elseif entity.thromTime <=960
      |             %witnessed and 6-16 hrs
      |             dist = EVT_DEFUSE3witnessed;
      |         else
      |             %witnessed and 16-24 hrs
      |             dist = EVT_DAWNwitnessed;
      |         end
      |     else
      |         dist = [];
      |     end
      | else
      |     if entity.outcomeType==1
      |         if entity.firstArrival <= 90
      |             dist = NT_90;
      |         elseif entity.firstArrival <= 180
      |             dist = NT_180;
      |         elseif entity.firstArrival <= 270
      |             dist = NT_270;
      |         else
      |             dist = NT_360;
      |         end
      |     elseif entity.outcomeType==2
      |         if entity.firstArrival <= 90
      |             dist = tPA_90;
      |         elseif entity.firstArrival <= 180
      |             dist = tPA_180;
      |         elseif entity.firstArrival <= 270
      |             dist = tPA_270;
      |         else
      |             dist = tPA_360;
      |         end
      |     else
      |         dist = [];
      |     end
      | end
      | if isempty(dist)
      |     entity.outcome = 999; %error message basically
      | else
      |     b = find(dist(:)<entity.randOutcome);
      |     if isempty(b)
      |         entity.outcome=0;
      |     else
      |         entity.outcome = b(length(b));
      |     end
      | end
  Yes : EntityTerminator  InputPortMessageModes=m  EntryAction=readTimer(entity.totalTime);  NumberEntitiesArrived=on
      settings: OutputPortMap=o0
  tPA Responsive?{,1,3,5} (4 alike) : EntityOutputSwitch  InputPortMessageModes=m  OutputPortMessageModes=m,m  SwitchingCriterion=From attribute  SwitchAttributeName=whichPort
  tPA Responsive?2 : EntityOutputSwitch  InputPortMessageModes=m  OutputPortMessageModes=m,m,m  NumberOutputPorts=3  SwitchingCriterion=From attribute  SwitchAttributeName=whichPort
      settings: OutputPortMap=o0,o1,o2
  tPA Responsive?4 : EntityOutputSwitch  InputPortMessageModes=m  OutputPortMessageModes=m,m,m  NumberOutputPorts=3  SwitchingCriterion=From attribute  SwitchAttributeName=whichPort
      settings: OutputPortMap=o0,o1,o2
  wires:
  to A/1 -> Travel to A/1
  Entity Terminator/1 -> End CSC/1
  CSC tPA/1 -> tPA Responsive?1/1
  CSC Throm/1 -> Merge Entry to CSC1/1
  tPA Responsive?1/1 -> Entity Multicast1/1
  Multicast Receive Queue/1 -> CSC Throm/1
  tPA Responsive?1/2 -> Merge Entry to CSC1/2
  Travel to A/1 -> tPA Responsive?2/1
  tPA Responsive?2/1 -> Entity Multicast2/1
  tPA Responsive?2/2 -> CSC tPA/1
  tPA Responsive?2/3 -> Merge Entry to CSC1/3
  Merge Entry to CSC1/1 -> Upgrade_A/1
  Upgrade_A/1 -> Entity Terminator/1
  tPA Responsive?3/1 -> Entity Multicast3/1
  tPA Responsive?4/3 -> Merge Entry to CSC2/3
  CSC Throm2/1 -> Merge Entry to CSC2/1
  tPA Responsive?4/2 -> CSC tPA2/1
  tPA Responsive?4/1 -> Entity Multicast4/1
  Merge Entry to CSC2/1 -> Upgrade_C/1
  tPA Responsive?3/2 -> Merge Entry to CSC2/2
  CSC tPA2/1 -> tPA Responsive?3/1
  Multicast Receive Queue1/1 -> CSC Throm2/1
  Entity Terminator1/1 -> End CSC1/1
  Travel to C/1 -> tPA Responsive?4/1
  Upgrade_C/1 -> Entity Terminator1/1
  PSC to CSC/1 -> Transfers/1
  Travel to B/1 -> PSC/1
  PSC to CSC/2 -> Entity Multicast/1
  PSC/1 -> tPA Responsive?/1
  tPA Responsive?/2 -> Upgrade_B/1
  Yes/1 -> End PSC/1
  Upgrade_B/1 -> Yes/1
  tPA Responsive?5/1 -> PSC to CSC/1
  PSC to CSC1/2 -> Entity Multicast5/1
  PSC to CSC1/1 -> Transfers1/1
  tPA Responsive?5/2 -> PSC to CSC1/1
  tPA Responsive?/1 -> Severity Marker1/1
  Severity Marker1/1 -> tPA Responsive?5/1
  to B/1 -> Travel to B/1
  to C/1 -> Travel to C/1
